simulink model "CruiseControlSK"  (R2022a)
settings: Solver=ode4  StartTime=0.0  StopTime=Tsim  FixedStep=Ts  RelTol=1e-3
values from neighbouring files (symbols this model uses):
  alfn = [40,25,16,12,10]    [CruiseControl.m]
  Beta = 0.4    [CruiseControl.m]
  Cambio = 5    [CruiseControl.m]
  Cr = 0.001    [CruiseControl.m]
  g = 9.8    [CruiseControl.m]
  I0 = Ue/Ki    (= 1.187)    [CruiseControl.m]
  Ka = (1/2)*rho*Cd*A    (= 0.4992)    [CruiseControl.m]
  Ki = 0.1    [CruiseControl.m]
  Kp = 0.5    [CruiseControl.m]
  Kperalte = Thetap/Td    (= 0.0261799387799)    [CruiseControl.m]
  m = 1200    [CruiseControl.m]    (also in ENCODER.m = 10)
  Omgm = 418.87    [CruiseControl.m]
  Tf = Ti+Td    (= 11)    [CruiseControl.m]
  Ti = 7    [CruiseControl.m]
  Tm = 200    [CruiseControl.m]
  V0 = 20    [CruiseControl.m]
settings Model: Creator=andres  LastModifiedBy=andres

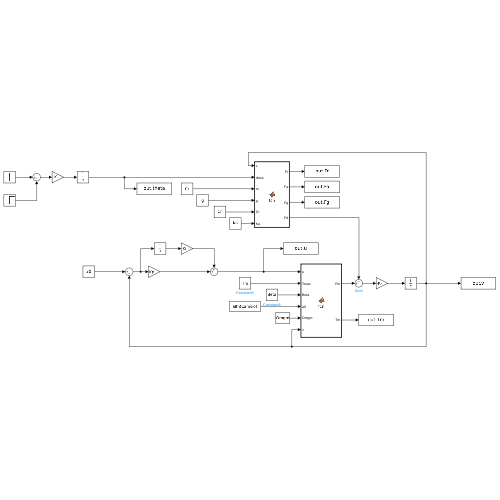
[thumbnail: Simulink's stored preview of the top-level diagram]
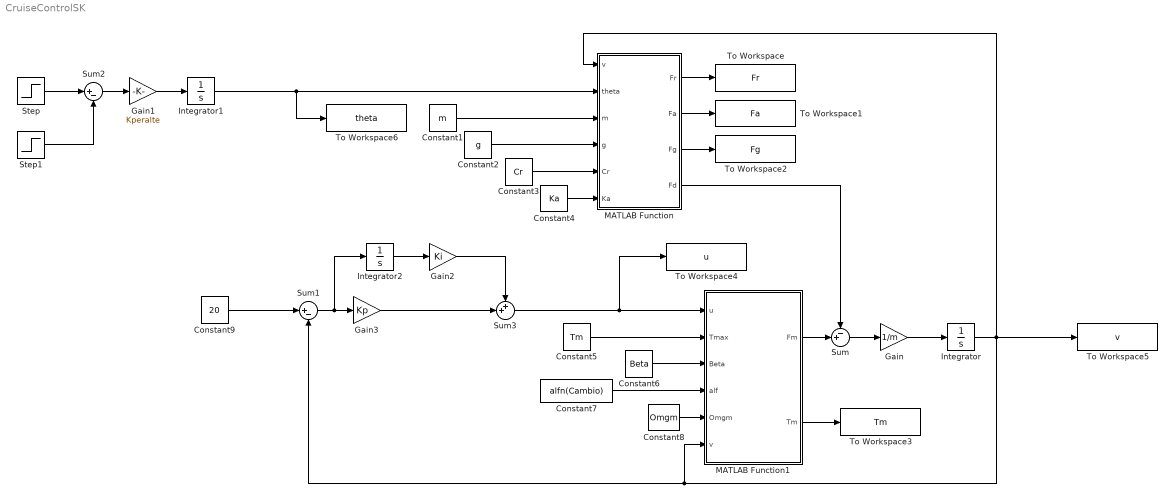
== system CruiseControlSK ==
  Constant1 : Constant  Value=m
  Constant2 : Constant  Value=g
  Constant3 : Constant  Value=Cr
  Constant4 : Constant  Value=Ka
  Constant5 : Constant  Value=Tm
  Constant6 : Constant  Value=Beta
  Constant7 : Constant  Value=alfn(Cambio)
  Constant8 : Constant  Value=Omgm
  Constant9 : Constant  Value=20
  Gain : Gain  Gain=1/m
  Gain1 : Gain  Gain=Kperalte
  Gain2 : Gain  Gain=Ki
  Gain3 : Gain  Gain=Kp
  Integrator : Integrator  InitialCondition=V0
  Integrator1 : Integrator
  Integrator2 : Integrator  InitialCondition=I0
  MATLAB Function : MATLAB Function  TreatAsAtomicUnit=on
  MATLAB Function1 : MATLAB Function  TreatAsAtomicUnit=on
  Step : Step  Time=Ti  SampleTime=0
  Step1 : Step  Time=Tf  SampleTime=0
  Sum : Sum  Inputs=-+|
  Sum1 : Sum  Inputs=|+-
  Sum2 : Sum  Inputs=|+-
  Sum3 : Sum  Inputs=++|
  To Workspace : ToWorkspace  VariableName=Fr  SaveFormat=Timeseries  SampleTime=-1
  To Workspace1 : ToWorkspace  VariableName=Fa  SaveFormat=Timeseries  SampleTime=-1
  To Workspace2 : ToWorkspace  VariableName=Fg  SaveFormat=Timeseries  SampleTime=-1
  To Workspace3 : ToWorkspace  VariableName=Tm  SaveFormat=Timeseries  SampleTime=-1
  To Workspace4 : ToWorkspace  VariableName=u  SaveFormat=Timeseries  SampleTime=-1
  To Workspace5 : ToWorkspace  VariableName=v  SaveFormat=Timeseries  SampleTime=-1
  To Workspace6 : ToWorkspace  VariableName=theta  SaveFormat=Timeseries  SampleTime=-1
  wires:
  Integrator/1 -> To Workspace5/1, Sum1/2, MATLAB Function1/6(v), MATLAB Function/1(v)
  MATLAB Function/1(Fr) -> To Workspace/1
  MATLAB Function/2(Fa) -> To Workspace1/1
  MATLAB Function/3(Fg) -> To Workspace2/1
  Integrator1/1 -> To Workspace6/1, MATLAB Function/2(theta)
  Constant1/1 -> MATLAB Function/3(m)
  Constant2/1 -> MATLAB Function/4(g)
  Constant3/1 -> MATLAB Function/5(Cr)
  Constant4/1 -> MATLAB Function/6(Ka)
  MATLAB Function/4(Fd) -> Sum/1
  MATLAB Function1/1(Fm) -> Sum/2
  Constant5/1 -> MATLAB Function1/2(Tmax)
  Constant6/1 -> MATLAB Function1/3(Beta)
  Constant7/1 -> MATLAB Function1/4(alf)
  Gain/1 -> Integrator/1
  Sum/1 -> Gain/1
  MATLAB Function1/2(Tm) -> To Workspace3/1
  Constant8/1 -> MATLAB Function1/5(Omgm)
  Sum1/1 -> Integrator2/1, Gain3/1
  Constant9/1 -> Sum1/1
  Step/1 -> Sum2/1
  Sum2/1 -> Gain1/1
  Step1/1 -> Sum2/2
  Gain1/1 -> Integrator1/1
  Gain3/1 -> Sum3/2
  Sum3/1 -> To Workspace4/1, MATLAB Function1/1(u)
  Integrator2/1 -> Gain2/1
  Gain2/1 -> Sum3/1

== matlab function CruiseControlSK/MATLAB Function1 ==
  data: u input; Tmax input; Beta input; alf input; Omgm input; v input; Fm output; Tm output
function [Fm, Tm] = fcn(u,Tmax,Beta,alf,Omgm,v)
    Tm=Tmax*(1-Beta*(alf*v/Omgm-1)^2);
    Fm=alf*u*Tm;
end

== matlab function CruiseControlSK/MATLAB Function ==
  data: v input; Fr output; theta input; m input; g input; Cr input; Ka input; Fa output; Fg output; Fd output
function [Fr, Fa , Fg , Fd] = fcn(v,theta,m,g,Cr,Ka)
  Fr=m*g*Cr*sign(v);
  Fa=Ka*v^2;
  Fg=m*g*sin(theta);
  Fd=Fr+Fa+Fg;
end
